simulink model "Simulazione_controllo"  (R2020a)
settings: Solver=VariableStepAuto  StartTime=0.0  StopTime=1000  RelTol=1e-3
values from neighbouring files (symbols this model uses):
  A = A_lin_eq    [Ascensione.m]    (also in Sistema.m; f_tilde.m = [-0.0014   -0.0000         0)
  Ad = sysD.a    [Ascensione.m]    (also in Sistema.m)
  B = B_lin_eq(:,1)    [Ascensione.m]    (also in Sistema.m; f_tilde.m = [0.0014)
  Bd = sysD.b    [Ascensione.m]    (also in Sistema.m)
  C = [0 1 0]    [Ascensione.m]    (also in Sistema.m)
  Ts = 0.05    [Ascensione.m]    (also in Sistema.m)
  x_0 = [0 0 0].'    [Pianificazione_senza_vincoli.m]
settings Model: Creator=andre  LastModifiedBy=andre
settings DebuggingCC: ArithmeticOperatorsInVariantConditions=warning
settings SFSimCC: CustomCodeUndefinedFunction=UseInterfaceOnly

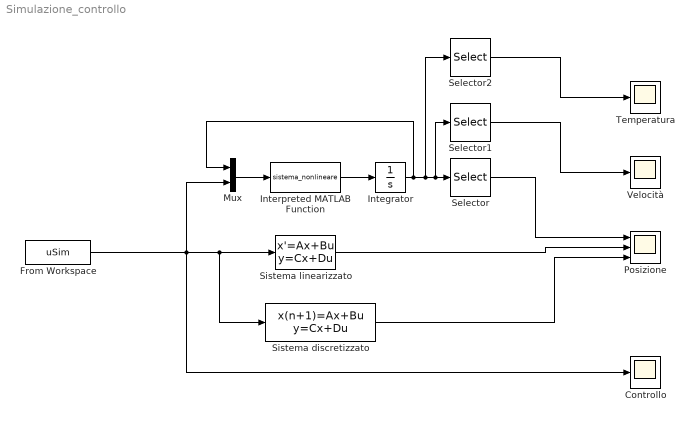
== system Simulazione_controllo ==
  Controllo : Scope
  From Workspace : FromWorkspace  VariableName=uSim  SampleTime=Ts  OutputAfterFinalValue=Holding final value
  Integrator : Integrator  InitialCondition=x_0
  Interpreted MATLAB Function : MATLABFcn  MATLABFcn=sistema_nonlineare
  Mux : Mux  Inputs=2
  Posizione : Scope  NumInputPorts=3
  Selector : Selector  InputPortWidth=3  IndexOptions=Index vector (dialog)  Indices=[2]  OutputSizes=1
  Selector1 : Selector  InputPortWidth=3  IndexOptions=Index vector (dialog)  Indices=[3]  OutputSizes=1
  Selector2 : Selector  InputPortWidth=3  IndexOptions=Index vector (dialog)  Indices=[1]  OutputSizes=1
  Sistema discretizzato : DiscreteStateSpace  A=Ad  B=Bd  C=C  D=0  InitialCondition=x_0  SampleTime=Ts
  Sistema linearizzato : StateSpace  A=A  B=B  C=C  D=0  InitialCondition=x_0
  Temperatura : Scope
  Velocità : Scope
  wires:
  Sistema linearizzato/1 -> Posizione/2
  From Workspace/1 -> Mux/2, Controllo/1, Sistema discretizzato/1, Sistema linearizzato/1
  Sistema discretizzato/1 -> Posizione/3
  Integrator/1 -> Mux/1, Selector2/1, Selector1/1, Selector/1
  Selector/1 -> Posizione/1
  Selector1/1 -> Velocità/1
  Mux/1 -> Interpreted MATLAB Function/1
  Interpreted MATLAB Function/1 -> Integrator/1
  Selector2/1 -> Temperatura/1
